simulink model "PD_grav"  (R2025b)
settings: Solver=VariableStepAuto  StartTime=0.0  StopTime=10.0  RelTol=1e-3
values from neighbouring files (symbols this model uses):
  alpha = 1    [FIREFIGHTER_AID.m]    (also in Setup_CSDR_Simulation.m = -1.57079632679; Setup_CSDR_Simulation_NL.m = -1.57079632679)
  D = [d1 0; 0 d2]    [Setup_CSDR_Simulation.m]    (also in Setup_CSDR_Simulation_NL.m)
  g = 1    [FIREFIGHTER_AID.m]    (also in Setup_CSDR_Simulation.m = 9.81; Setup_CSDR_Simulation_NL.m = 9.81)
  I1 = 1.5    [Setup_CSDR_Simulation.m]    (also in Setup_CSDR_Simulation_NL.m)
  I2 = 0.5    [Setup_CSDR_Simulation.m]    (also in Setup_CSDR_Simulation_NL.m)
  kd = [7.92 0 ... (first row only)    [Setup_CSDR_Simulation_NL.m]
  kp = [1.78 0 ... (first row only)    [Setup_CSDR_Simulation_NL.m]
  l_c1 = 1    [FIREFIGHTER_AID.m]    (also in Setup_CSDR_Simulation.m = 0.5; Setup_CSDR_Simulation_NL.m = 0.5)
  m1 = 1    [FIREFIGHTER_AID.m]    (also in Setup_CSDR_Simulation.m = 15; Setup_CSDR_Simulation_NL.m = 15)
  m2 = 1    [FIREFIGHTER_AID.m]    (also in Setup_CSDR_Simulation.m = 8; Setup_CSDR_Simulation_NL.m = 8)
  S = eye(2)    [Setup_CSDR_Simulation.m]    (also in Setup_CSDR_Simulation_NL.m)
settings Model: Creator=vladm  LastModifiedBy=vladm

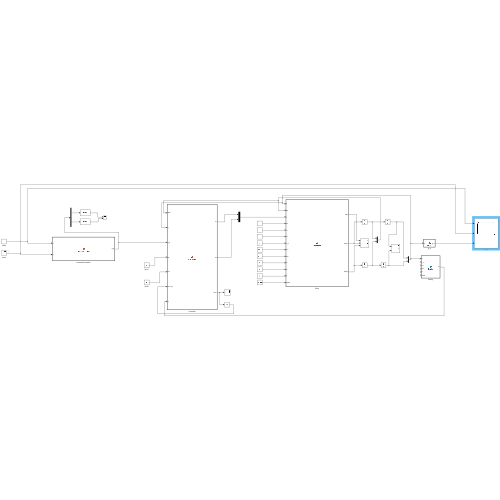
[thumbnail: Simulink's stored preview of the top-level diagram]
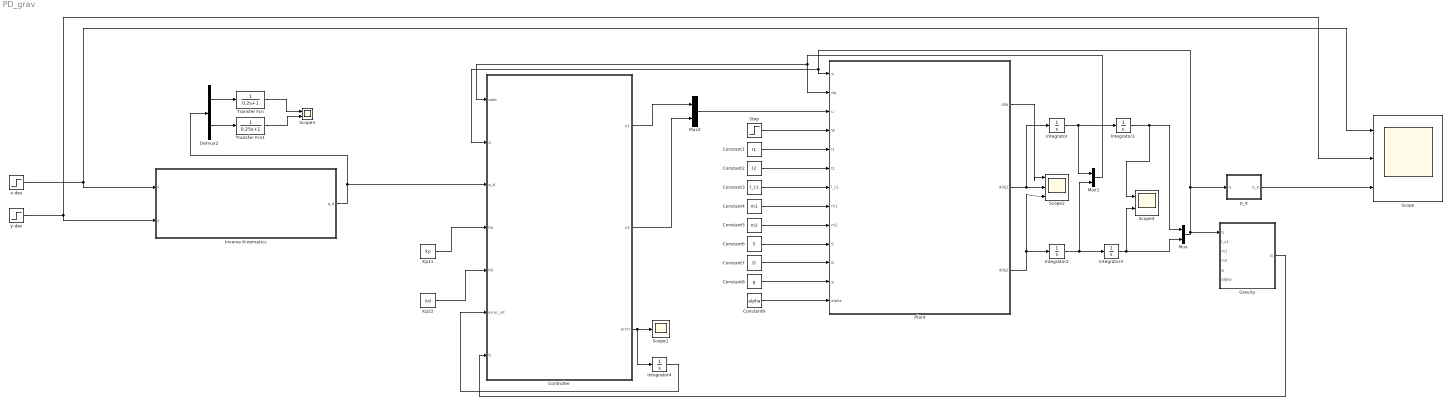
== system PD_grav ==
  Constant1 : Constant  Value=I1
  Constant2 : Constant  Value=I2
  Constant3 : Constant  Value=l_c1
  Constant4 : Constant  Value=m1
  Constant5 : Constant  Value=m2
  Constant6 : Constant  Value=S
  Constant7 : Constant  Value=D
  Constant8 : Constant  Value=g
  Constant9 : Constant  Value=alpha
  Controller : MATLAB Function  TreatAsAtomicUnit=on
  Demux2 : Demux  Outputs=2
  Gravity : MATLAB Function  TreatAsAtomicUnit=on
  Integrator{,1..4} (5 alike) : Integrator
  Inverse Kinematics : MATLAB Function  TreatAsAtomicUnit=on
  Kp11 : Constant  Value=kp  VectorParams1D=off
  Kp22 : Constant  Value=kd  VectorParams1D=off
  Mux : Mux  Inputs=2
  Mux1 : Mux  Inputs=2
  Mux2 : Mux  Inputs=2
  Plant : MATLAB Function  TreatAsAtomicUnit=on
  Scope : Scope  NumInputPorts=3
      settings: ActiveDisplayYMinimum=-1.2944523033330551  ActiveDisplayYMaximum=1.9782394646233648
  Scope1 : Scope
      settings: ActiveDisplayYMinimum=-1.4149117676445186  ActiveDisplayYMaximum=1.7230412328364795
  Scope2 : Scope  NumInputPorts=3
      settings: ActiveDisplayYMinimum=-356.26643794331915  ActiveDisplayYMaximum=879.81756407161015  DataLoggingVariableName=ScopeData2
  Scope3 : Scope  NumInputPorts=2
      settings: ActiveDisplayYMinimum=-0.49677109192679447  ActiveDisplayYMaximum=3.5520445414854449  DataLoggingVariableName=ScopeData3
  Scope4 : Scope  NumInputPorts=2
      settings: ActiveDisplayYMinimum=0.91734967521944688  ActiveDisplayYMaximum=0.94190036964998114  DataLoggingVariableName=ScopeData4
  Step : Step  Time=20  After=[0;0]  SampleTime=0
  Transfer Fcn : TransferFcn  Denominator=[0.2 1]
  Transfer Fcn1 : TransferFcn  Denominator=[0.25 1]
  p_e : MATLAB Function  TreatAsAtomicUnit=on
  x-des : Step  Time=2  After=0.985  SampleTime=0
  y-des : Step  Time=2  After=0.174  SampleTime=0
  wires:
  Plant/2(ddq1) -> Integrator/1, Scope2/2
  y-des/1 -> Inverse Kinematics/2(y), Scope/2
  x-des/1 -> Inverse Kinematics/1(x), Scope/1
  Step/1 -> Plant/4(W)
  Constant1/1 -> Plant/5(I1)
  Constant2/1 -> Plant/6(I2)
  Constant3/1 -> Plant/7(l_c1)
  Constant4/1 -> Plant/8(m1)
  Constant5/1 -> Plant/9(m2)
  Constant6/1 -> Plant/10(S)
  Constant7/1 -> Plant/11(D)
  Constant8/1 -> Plant/12(g)
  Constant9/1 -> Plant/13(alpha)
  Kp11/1 -> Controller/4(Kp)
  p_e/1(p_e) -> Scope/3
  Integrator1/1 -> Scope4/1, Mux/1
  Integrator/1 -> Mux1/1, Integrator1/1
  Kp22/1 -> Controller/5(Kd)
  Demux2/1 -> Transfer Fcn/1
  Inverse Kinematics/1(q_d) -> Demux2/1, Controller/3(q_d)
  Gravity/1(G) -> Controller/7(G)
  Plant/3(ddq2) -> Scope2/3, Integrator2/1
  Integrator2/1 -> Mux1/2, Integrator3/1
  Mux/1 -> p_e/1(q), Controller/2(q), Plant/1(q), Gravity/1(q)
  Integrator3/1 -> Mux/2, Scope4/2
  Mux1/1 -> Plant/2(dq), Controller/1(qdot)
  Controller/1(u1) -> Mux2/1
  Controller/2(u2) -> Mux2/2
  Mux2/1 -> Plant/3(u)
  Controller/3(error) -> Integrator4/1, Scope1/1
  Transfer Fcn/1 -> Scope3/1
  Demux2/2 -> Transfer Fcn1/1
  Transfer Fcn1/1 -> Scope3/2
  Plant/1(ddq) -> Scope2/1
  Integrator4/1 -> Controller/6(error_int)

== matlab function PD_grav/Controller ==
  data: qdot input; q input; q_d input; u1 output; Kp input; Kd input; error_int input; G input; u2 output; error output
function [u1, u2, error] = NLcontrol(qdot, q, q_d, Kp, Kd,error_int, G)
    %u = kp*e - kd*qdot + g(q)
    Ki = [10 0; 0 10];
    error = q_d-q; 
    u = Kp*error + Ki*error_int - Kd*qdot + G;
    u1=u(1);
    u2=u(2);

== matlab function PD_grav/Inverse Kinematics ==
  data: x input; q_d output; y input
function q_d  = InverseKinematics(x, y)
    % This block runs every time step
    
    % Extension (Prismatic Joint)
    q2_d = sqrt(x^2 + y^2);
    
    % Rotation (Revolute Joint)
    % We use atan2 to handle all quadrants automatically
    q1_d = atan2(y, x);

    q_d = [q1_d; q2_d];
end

== matlab function PD_grav/Plant ==
  data: ddq output; q input size=2 1; dq input size=2 1; u input; ddq1 output; W input; I1 input; I2 input; l_c1 input; m1 input; m2 input; S input; D input; g input; alpha input; ddq2 output
function [ddq,ddq1, ddq2]   = PolarRobot(q, dq, u, W, I1, I2, l_c1, m1, m2, S, D, g, alpha)
% Only the dynamic equations remain here

% Vectors
% M(q) - Mass matrix (Changes with q2)
M = [I1 + I2 + (l_c1^2)*m1 + m2*(q(2)^2), 0;
     0, m2];

% c(q,dq) - Coriolis (Changes with q2, dq1, dq2)
c = [2*dq(1)*dq(2)*m2*q(2);
    -(dq(1)^2)*m2*q(2)];

% G(q) - Gravity (Changes with q1, q2)
G = [g*cos(alpha - q(1))*(l_c1*m1 + m2*q(2));
    -g*m2*sin(alpha - q(1))];

% J(q) - Jacobian
J = [-q(2)*sin(q(1)), cos(q(1));
      q(2)*cos(q(1)), sin(q(1))];

invertedM = inv(M);
% Solving for ddq
ddq = invertedM*(S*u+J'*W-c-D*dq-G);
ddq1 = ddq(1);
ddq2 = ddq(2);

== matlab function PD_grav/p_e ==
  data: q input size=2 1; p_e output size=2 1
function p_e = ee_p(q)

p_e = [q(2)*cos(q(1)); q(2)*sin(q(1))];

== matlab function PD_grav/Gravity ==
  data: q input size=2 1; G output; l_c1 input; m1 input; m2 input; g input; alpha input
function  G    = Gravity(q, l_c1, m1, m2, g, alpha)
% Only the dynamic equations remain here

% G(q) - Gravity (Changes with q1, q2)
G = [g*cos(alpha - q(1))*(l_c1*m1 + m2*q(2));
    -g*m2*sin(alpha - q(1))];
